simulink model "sim"  (R2024a)
settings: Solver=VariableStepAuto  StartTime=0.0  StopTime=500  RelTol=1e-3
undefined symbols (not defined in the file): den_pp, Kr, num_pp
settings Model: Creator=grabo  LastModifiedBy=grabo

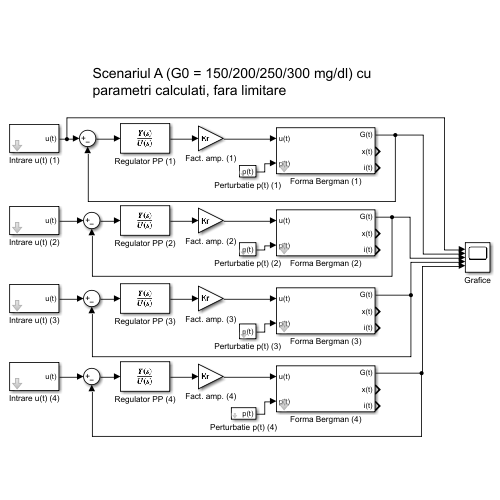
[thumbnail: Simulink's stored preview of the top-level diagram]
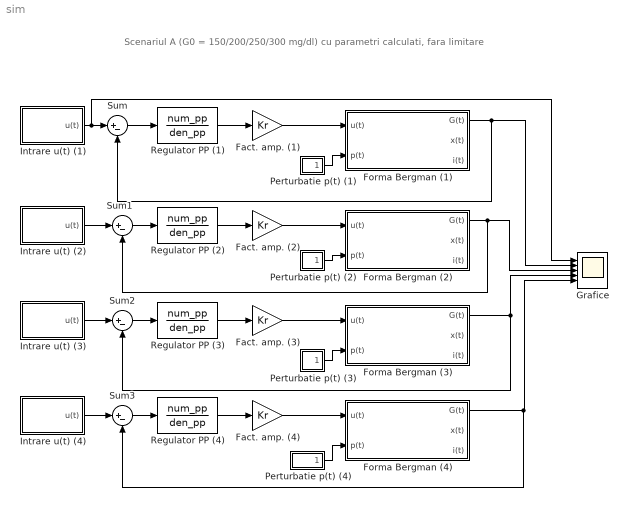
== system sim ==
  note: Scenariul A (G0 = 150/200/250/300 mg/dl) cu parametri calculati, fara limitare
  Fact. amp. (1) : Gain  Gain=Kr
  Fact. amp. (2) : Gain  Gain=Kr
  Fact. amp. (3) : Gain  Gain=Kr
  Fact. amp. (4) : Gain  Gain=Kr
  Forma Bergman (1) : Subsystem  mask{V=120, Gb=80, p1=0.019, p2=0.021, p3=10.19*10^(-6), n=0.177, G0=150}
      mask prompts: V "V ="; Gb "Gb ="; p1 "p1 ="; p2 "p2 ="; p3 "p3 ="; n "n ="; G0 "G0 ="
  Forma Bergman (2) : Subsystem  mask{V=120, Gb=80, p1=0.019, p2=0.021, p3=10.19*10^(-6), n=0.177, G0=200}
      mask prompts: V "V ="; Gb "Gb ="; p1 "p1 ="; p2 "p2 ="; p3 "p3 ="; n "n ="; G0 "G0 ="
  Forma Bergman (3) : Subsystem  mask{V=120, Gb=80, p1=0.019, p2=0.021, p3=10.19*10^(-6), n=0.177, G0=250}
      mask prompts: V "V ="; Gb "Gb ="; p1 "p1 ="; p2 "p2 ="; p3 "p3 ="; n "n ="; G0 "G0 ="
  Forma Bergman (4) : Subsystem  mask{V=120, Gb=80, p1=0.019, p2=0.021, p3=10.19*10^(-6), n=0.177, G0=300}
      mask prompts: V "V ="; Gb "Gb ="; p1 "p1 ="; p2 "p2 ="; p3 "p3 ="; n "n ="; G0 "G0 ="
  Grafice : Scope  NumInputPorts=5
  Intrare u(t) (1) : Subsystem  mask{With_u=1, Gref=80}
      mask prompts: With_u "With_u ="; Gref "Gref ="
  Intrare u(t) (2) : Subsystem  mask{With_u=1, Gref=80}
      mask prompts: With_u "With_u ="; Gref "Gref ="
  Intrare u(t) (3) : Subsystem  mask{With_u=1, Gref=80}
      mask prompts: With_u "With_u ="; Gref "Gref ="
  Intrare u(t) (4) : Subsystem  mask{With_u=1, Gref=80}
      mask prompts: With_u "With_u ="; Gref "Gref ="
  Perturbatie p(t) (1) : Subsystem  mask{Dg=10*10^3, Ag=0.8, tgM=40, With_p=0}
      mask prompts: Dg "Dg ="; Ag "Ag ="; tgM "tgM ="; With_p "With_p ="
  Perturbatie p(t) (2) : Subsystem  mask{Dg=10*10^3, Ag=0.8, tgM=40, With_p=0}
      mask prompts: Dg "Dg ="; Ag "Ag ="; tgM "tgM ="; With_p "With_p ="
  Perturbatie p(t) (3) : Subsystem  mask{Dg=10*10^3, Ag=0.8, tgM=40, With_p=0}
      mask prompts: Dg "Dg ="; Ag "Ag ="; tgM "tgM ="; With_p "With_p ="
  Perturbatie p(t) (4) : Subsystem  mask{Dg=10*10^3, Ag=0.8, tgM=40, With_p=0}
      mask prompts: Dg "Dg ="; Ag "Ag ="; tgM "tgM ="; With_p "With_p ="
  Regulator PP (1) : TransferFcn  Numerator=num_pp  Denominator=den_pp
  Regulator PP (2) : TransferFcn  Numerator=num_pp  Denominator=den_pp
  Regulator PP (3) : TransferFcn  Numerator=num_pp  Denominator=den_pp
  Regulator PP (4) : TransferFcn  Numerator=num_pp  Denominator=den_pp
  Sum{,1..3} (4 alike) : Sum  Inputs=|+-
  wires:
  Perturbatie p(t) (1)/1(p(t)) -> Forma Bergman (1)/2(p(t))
  Forma Bergman (2)/1(G(t)) -> Sum1/2, Grafice/3
  Forma Bergman (3)/1(G(t)) -> Grafice/4, Sum2/2
  Perturbatie p(t) (2)/1(p(t)) -> Forma Bergman (2)/2(p(t))
  Forma Bergman (1)/1(G(t)) -> Grafice/2, Sum/2
  Forma Bergman (4)/1(G(t)) -> Sum3/2, Grafice/5
  Perturbatie p(t) (3)/1(p(t)) -> Forma Bergman (3)/2(p(t))
  Perturbatie p(t) (4)/1(p(t)) -> Forma Bergman (4)/2(p(t))
  Regulator PP (1)/1 -> Fact. amp. (1)/1
  Intrare u(t) (1)/1(u(t)) -> Grafice/1, Sum/1
  Sum1/1 -> Regulator PP (2)/1
  Sum2/1 -> Regulator PP (3)/1
  Intrare u(t) (3)/1(u(t)) -> Sum2/1
  Intrare u(t) (4)/1(u(t)) -> Sum3/1
  Intrare u(t) (2)/1(u(t)) -> Sum1/1
  Sum/1 -> Regulator PP (1)/1
  Regulator PP (2)/1 -> Fact. amp. (2)/1
  Regulator PP (3)/1 -> Fact. amp. (3)/1
  Regulator PP (4)/1 -> Fact. amp. (4)/1
  Fact. amp. (4)/1 -> Forma Bergman (4)/1(u(t))
  Fact. amp. (2)/1 -> Forma Bergman (2)/1(u(t))
  Fact. amp. (1)/1 -> Forma Bergman (1)/1(u(t))
  Sum3/1 -> Regulator PP (4)/1
  Fact. amp. (3)/1 -> Forma Bergman (3)/1(u(t))

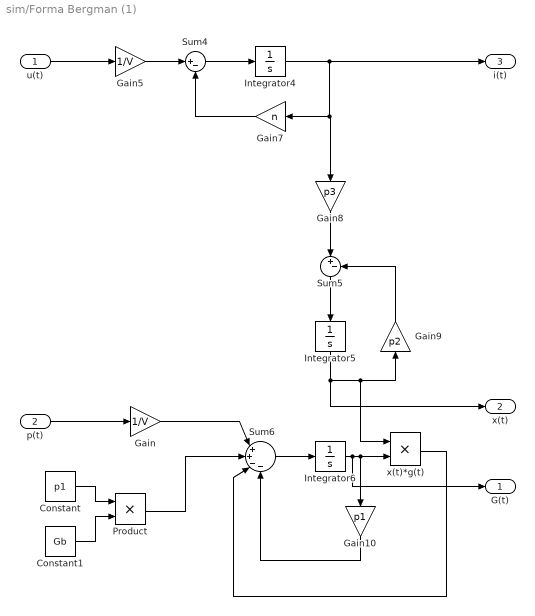
== system sim/Forma Bergman (1) ==
  u(t) : Inport
  p(t) : Inport  Port=2
  Constant : Constant  Value=p1
  Constant1 : Constant  Value=Gb
  Gain : Gain  Gain=1/V
  Gain10 : Gain  Gain=p1
  Gain5 : Gain  Gain=1/V
  Gain7 : Gain  Gain=n
  Gain8 : Gain  Gain=p3
  Gain9 : Gain  Gain=p2
  Integrator4 : Integrator
  Integrator5 : Integrator
  Integrator6 : Integrator  InitialCondition=G0
  Product : Product
  Sum4 : Sum  Inputs=|+-
  Sum5 : Sum  Inputs=|+-
  Sum6 : Sum  Inputs=|++--
  x(t)*g(t) : Product
  G(t) : Outport
  x(t) : Outport  Port=2
  i(t) : Outport  Port=3
  wires:
  Sum4/1 -> Integrator4/1
  Gain7/1 -> Sum4/2
  Integrator4/1 -> Gain7/1, Gain8/1, i(t)/1
  Gain8/1 -> Sum5/1
  Sum5/1 -> Integrator5/1
  Gain9/1 -> Sum5/2
  Sum6/1 -> Integrator6/1
  Integrator6/1 -> G(t)/1, Gain10/1, x(t)*g(t)/2
  Gain10/1 -> Sum6/4
  x(t)*g(t)/1 -> Sum6/3
  Product/1 -> Sum6/2
  Integrator5/1 -> x(t)/1, x(t)*g(t)/1, Gain9/1
  Gain5/1 -> Sum4/1
  u(t)/1 -> Gain5/1
  p(t)/1 -> Gain/1
  Gain/1 -> Sum6/1
  Constant/1 -> Product/1
  Constant1/1 -> Product/2

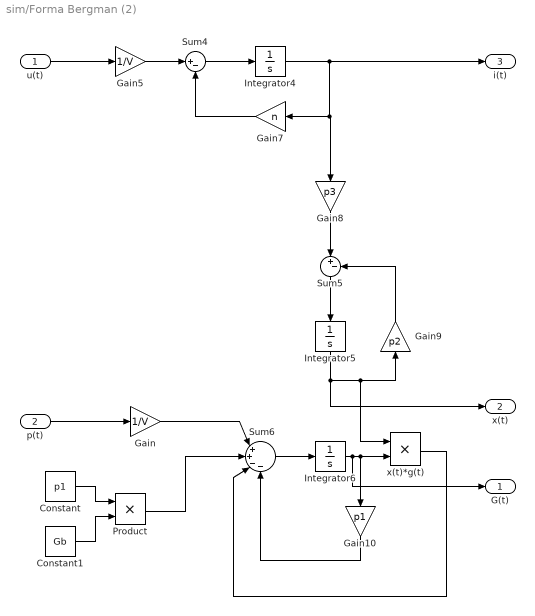
== system sim/Forma Bergman (2) ==
  u(t) : Inport
  p(t) : Inport  Port=2
  Constant : Constant  Value=p1
  Constant1 : Constant  Value=Gb
  Gain : Gain  Gain=1/V
  Gain10 : Gain  Gain=p1
  Gain5 : Gain  Gain=1/V
  Gain7 : Gain  Gain=n
  Gain8 : Gain  Gain=p3
  Gain9 : Gain  Gain=p2
  Integrator4 : Integrator
  Integrator5 : Integrator
  Integrator6 : Integrator  InitialCondition=G0
  Product : Product
  Sum4 : Sum  Inputs=|+-
  Sum5 : Sum  Inputs=|+-
  Sum6 : Sum  Inputs=|++--
  x(t)*g(t) : Product
  G(t) : Outport
  x(t) : Outport  Port=2
  i(t) : Outport  Port=3
  wires:
  Sum4/1 -> Integrator4/1
  Gain7/1 -> Sum4/2
  Integrator4/1 -> Gain7/1, Gain8/1, i(t)/1
  Gain8/1 -> Sum5/1
  Sum5/1 -> Integrator5/1
  Gain9/1 -> Sum5/2
  Sum6/1 -> Integrator6/1
  Integrator6/1 -> G(t)/1, Gain10/1, x(t)*g(t)/2
  Gain10/1 -> Sum6/4
  x(t)*g(t)/1 -> Sum6/3
  Product/1 -> Sum6/2
  Integrator5/1 -> x(t)/1, x(t)*g(t)/1, Gain9/1
  Gain5/1 -> Sum4/1
  u(t)/1 -> Gain5/1
  p(t)/1 -> Gain/1
  Gain/1 -> Sum6/1
  Constant/1 -> Product/1
  Constant1/1 -> Product/2

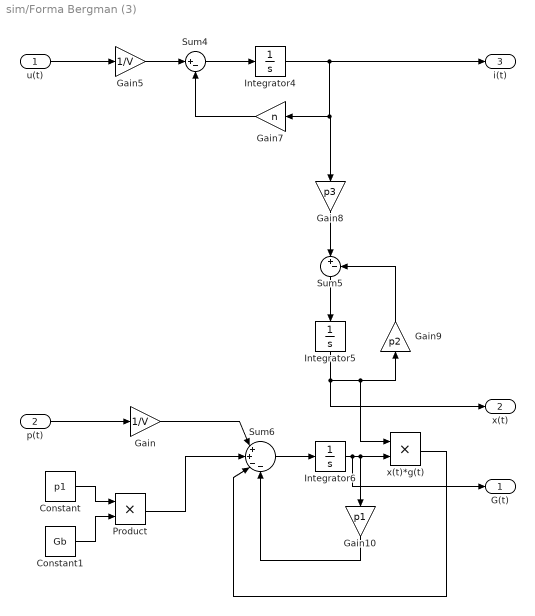
== system sim/Forma Bergman (3) ==
  u(t) : Inport
  p(t) : Inport  Port=2
  Constant : Constant  Value=p1
  Constant1 : Constant  Value=Gb
  Gain : Gain  Gain=1/V
  Gain10 : Gain  Gain=p1
  Gain5 : Gain  Gain=1/V
  Gain7 : Gain  Gain=n
  Gain8 : Gain  Gain=p3
  Gain9 : Gain  Gain=p2
  Integrator4 : Integrator
  Integrator5 : Integrator
  Integrator6 : Integrator  InitialCondition=G0
  Product : Product
  Sum4 : Sum  Inputs=|+-
  Sum5 : Sum  Inputs=|+-
  Sum6 : Sum  Inputs=|++--
  x(t)*g(t) : Product
  G(t) : Outport
  x(t) : Outport  Port=2
  i(t) : Outport  Port=3
  wires:
  Sum4/1 -> Integrator4/1
  Gain7/1 -> Sum4/2
  Integrator4/1 -> Gain7/1, Gain8/1, i(t)/1
  Gain8/1 -> Sum5/1
  Sum5/1 -> Integrator5/1
  Gain9/1 -> Sum5/2
  Sum6/1 -> Integrator6/1
  Integrator6/1 -> G(t)/1, Gain10/1, x(t)*g(t)/2
  Gain10/1 -> Sum6/4
  x(t)*g(t)/1 -> Sum6/3
  Product/1 -> Sum6/2
  Integrator5/1 -> x(t)/1, x(t)*g(t)/1, Gain9/1
  Gain5/1 -> Sum4/1
  u(t)/1 -> Gain5/1
  p(t)/1 -> Gain/1
  Gain/1 -> Sum6/1
  Constant/1 -> Product/1
  Constant1/1 -> Product/2

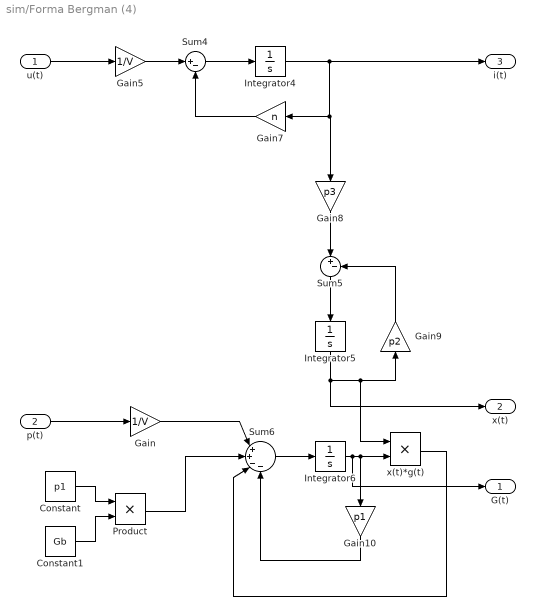
== system sim/Forma Bergman (4) ==
  u(t) : Inport
  p(t) : Inport  Port=2
  Constant : Constant  Value=p1
  Constant1 : Constant  Value=Gb
  Gain : Gain  Gain=1/V
  Gain10 : Gain  Gain=p1
  Gain5 : Gain  Gain=1/V
  Gain7 : Gain  Gain=n
  Gain8 : Gain  Gain=p3
  Gain9 : Gain  Gain=p2
  Integrator4 : Integrator
  Integrator5 : Integrator
  Integrator6 : Integrator  InitialCondition=G0
  Product : Product
  Sum4 : Sum  Inputs=|+-
  Sum5 : Sum  Inputs=|+-
  Sum6 : Sum  Inputs=|++--
  x(t)*g(t) : Product
  G(t) : Outport
  x(t) : Outport  Port=2
  i(t) : Outport  Port=3
  wires:
  Sum4/1 -> Integrator4/1
  Gain7/1 -> Sum4/2
  Integrator4/1 -> Gain7/1, Gain8/1, i(t)/1
  Gain8/1 -> Sum5/1
  Sum5/1 -> Integrator5/1
  Gain9/1 -> Sum5/2
  Sum6/1 -> Integrator6/1
  Integrator6/1 -> G(t)/1, Gain10/1, x(t)*g(t)/2
  Gain10/1 -> Sum6/4
  x(t)*g(t)/1 -> Sum6/3
  Product/1 -> Sum6/2
  Integrator5/1 -> x(t)/1, x(t)*g(t)/1, Gain9/1
  Gain5/1 -> Sum4/1
  u(t)/1 -> Gain5/1
  p(t)/1 -> Gain/1
  Gain/1 -> Sum6/1
  Constant/1 -> Product/1
  Constant1/1 -> Product/2

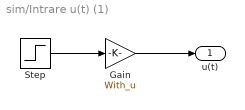
== system sim/Intrare u(t) (1) ==
  Gain : Gain  Gain=With_u
  Step : Step  Time=0  After=Gref  SampleTime=0
  u(t) : Outport
  wires:
  Step/1 -> Gain/1
  Gain/1 -> u(t)/1

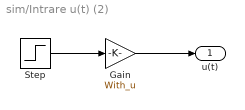
== system sim/Intrare u(t) (2) ==
  Gain : Gain  Gain=With_u
  Step : Step  Time=0  After=Gref  SampleTime=0
  u(t) : Outport
  wires:
  Step/1 -> Gain/1
  Gain/1 -> u(t)/1

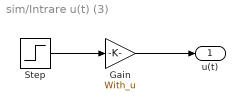
== system sim/Intrare u(t) (3) ==
  Gain : Gain  Gain=With_u
  Step : Step  Time=0  After=Gref  SampleTime=0
  u(t) : Outport
  wires:
  Step/1 -> Gain/1
  Gain/1 -> u(t)/1

== system sim/Intrare u(t) (4) ==
  Gain : Gain  Gain=With_u
  Step : Step  Time=0  After=Gref  SampleTime=0
  u(t) : Outport
  wires:
  Step/1 -> Gain/1
  Gain/1 -> u(t)/1

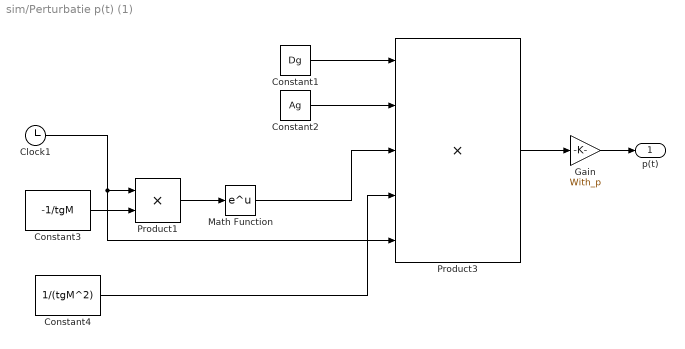
== system sim/Perturbatie p(t) (1) ==
  Clock1 : Clock
  Constant1 : Constant  Value=Dg
  Constant2 : Constant  Value=Ag
  Constant3 : Constant  Value=-1/tgM
  Constant4 : Constant  Value=1/(tgM^2)
  Gain : Gain  Gain=With_p
  Math Function : Math  SignedPower=on
  Product1 : Product
  Product3 : Product  Inputs=5
  p(t) : Outport
  wires:
  Clock1/1 -> Product3/5, Product1/1
  Constant3/1 -> Product1/2
  Product1/1 -> Math Function/1
  Constant4/1 -> Product3/4
  Constant1/1 -> Product3/1
  Constant2/1 -> Product3/2
  Math Function/1 -> Product3/3
  Product3/1 -> Gain/1
  Gain/1 -> p(t)/1

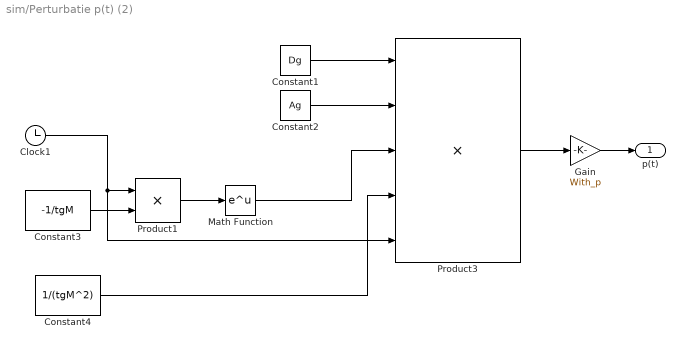
== system sim/Perturbatie p(t) (2) ==
  Clock1 : Clock
  Constant1 : Constant  Value=Dg
  Constant2 : Constant  Value=Ag
  Constant3 : Constant  Value=-1/tgM
  Constant4 : Constant  Value=1/(tgM^2)
  Gain : Gain  Gain=With_p
  Math Function : Math  SignedPower=on
  Product1 : Product
  Product3 : Product  Inputs=5
  p(t) : Outport
  wires:
  Clock1/1 -> Product3/5, Product1/1
  Constant3/1 -> Product1/2
  Product1/1 -> Math Function/1
  Constant4/1 -> Product3/4
  Constant1/1 -> Product3/1
  Constant2/1 -> Product3/2
  Math Function/1 -> Product3/3
  Product3/1 -> Gain/1
  Gain/1 -> p(t)/1

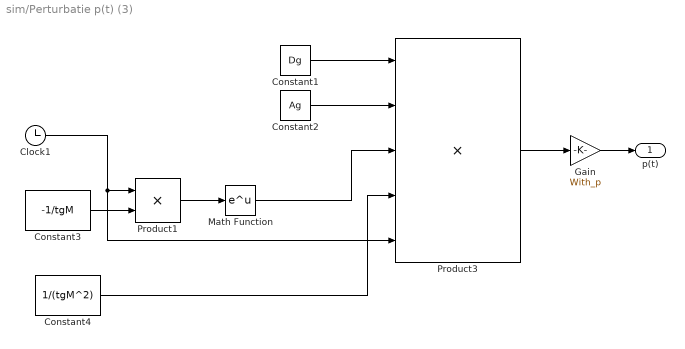
== system sim/Perturbatie p(t) (3) ==
  Clock1 : Clock
  Constant1 : Constant  Value=Dg
  Constant2 : Constant  Value=Ag
  Constant3 : Constant  Value=-1/tgM
  Constant4 : Constant  Value=1/(tgM^2)
  Gain : Gain  Gain=With_p
  Math Function : Math  SignedPower=on
  Product1 : Product
  Product3 : Product  Inputs=5
  p(t) : Outport
  wires:
  Clock1/1 -> Product3/5, Product1/1
  Constant3/1 -> Product1/2
  Product1/1 -> Math Function/1
  Constant4/1 -> Product3/4
  Constant1/1 -> Product3/1
  Constant2/1 -> Product3/2
  Math Function/1 -> Product3/3
  Product3/1 -> Gain/1
  Gain/1 -> p(t)/1

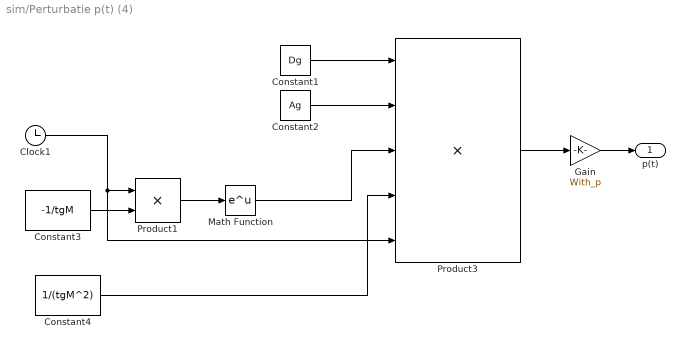
== system sim/Perturbatie p(t) (4) ==
  Clock1 : Clock
  Constant1 : Constant  Value=Dg
  Constant2 : Constant  Value=Ag
  Constant3 : Constant  Value=-1/tgM
  Constant4 : Constant  Value=1/(tgM^2)
  Gain : Gain  Gain=With_p
  Math Function : Math  SignedPower=on
  Product1 : Product
  Product3 : Product  Inputs=5
  p(t) : Outport
  wires:
  Clock1/1 -> Product3/5, Product1/1
  Constant3/1 -> Product1/2
  Product1/1 -> Math Function/1
  Constant4/1 -> Product3/4
  Constant1/1 -> Product3/1
  Constant2/1 -> Product3/2
  Math Function/1 -> Product3/3
  Product3/1 -> Gain/1
  Gain/1 -> p(t)/1
